simulink model "UDP_Send"  (R2023a)
settings: Solver=VariableStepAuto  StartTime=0.0  StopTime=Inf  RelTol=1e-3
libraries: instrumentlib x1
settings Model: Creator=pablo.gamboa  LastModifiedBy=pablo.gamboa

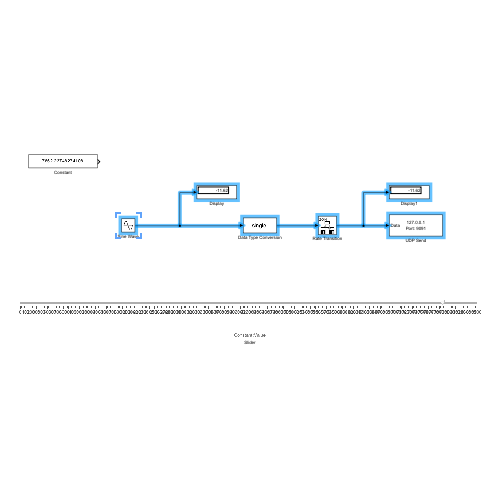
[thumbnail: Simulink's stored preview of the top-level diagram]
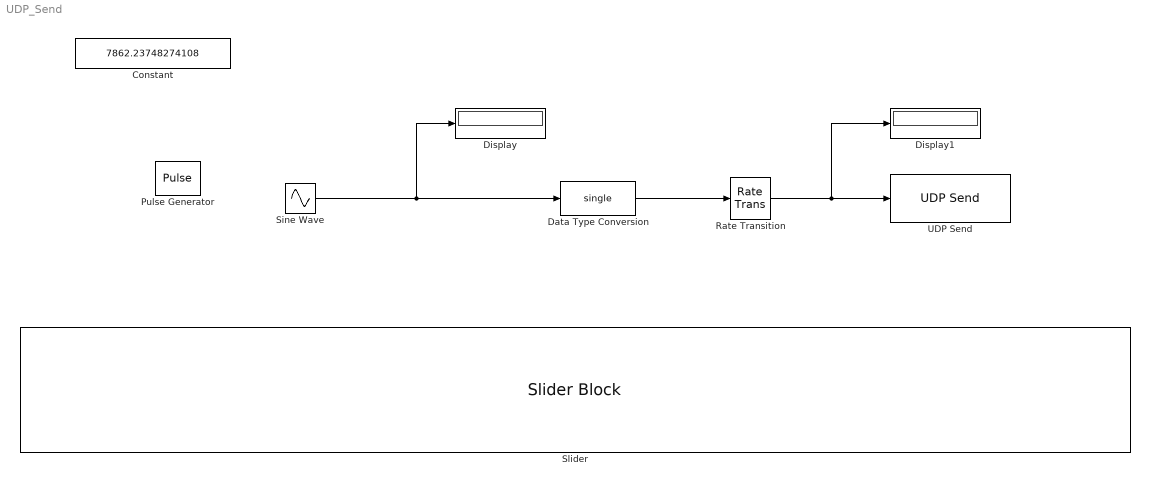
== system UDP_Send ==
  Constant : Constant  Value=7862.23748274108
  Data Type Conversion : DataTypeConversion  OutDataTypeStr=single  SaturateOnIntegerOverflow=off  RndMeth=Floor
  Display : Display
  Display1 : Display
  Rate Transition : RateTransition  OutPortSampleTime=0.1
  Sine Wave : Sin  Amplitude=1000  SampleTime=0
  Slider : SliderBlock  LabelPosition=Bottom  ScaleMax=8500  TickInterval=100
  UDP Send : instrumentlib/UDP Send  Host=127.0.0.1  Port=9091  LocalAddress=0.0.0.0  LocalPort=-1  EnablePortSharing=off  OutputDatagramPacketSize=512  ByteOrder=little-endian  EnableBlockingMode=off  SimulateUsing=Interpreted execution
  Pulse Generator : DiscretePulseGenerator  IOType=siggen  PulseType=Time based  PulseWidth=50
  wires:
  Data Type Conversion/1 -> Rate Transition/1
  Rate Transition/1 -> Display1/1, UDP Send/1
  Sine Wave/1 -> Display/1, Data Type Conversion/1
